simulink model "tarea"  (Simulink 7.5)
settings: Solver=ode4  StartTime=0.0  StopTime=20  FixedStep=.0001  RelTol=1e-3
values from neighbouring files (symbols this model uses):
  K1 = 3.06    [parametros.m]
  K2 = -0.7160    (= -0.716)    [parametros.m]
  L1 = 2*zo*wno-ka/(m*l)    (= 35.8260869565)    [parametros.m]
  L2 = wno^2-L1*ka/(m*l)-g/l    (= 275.117202268)    [parametros.m]
undefined symbols (not defined in the file or in its folder): G, Ka, L, M
settings Model: Creator=Lalo  LastModifiedBy=Lalo
settings OptimizationCC: ExpressionDepthLimit=128
settings DebuggingCC: UnderspecifiedInitializationDetection=Simplified  FcnCallInpInsideContextMsg=Enable All  StateNameClashWarn=none
settings CodeAppCC: CustomSymbolStrType=$N$R$M_T
settings GRTTargetCC: TargetFunctionLibrary=C89/C90 (ANSI)

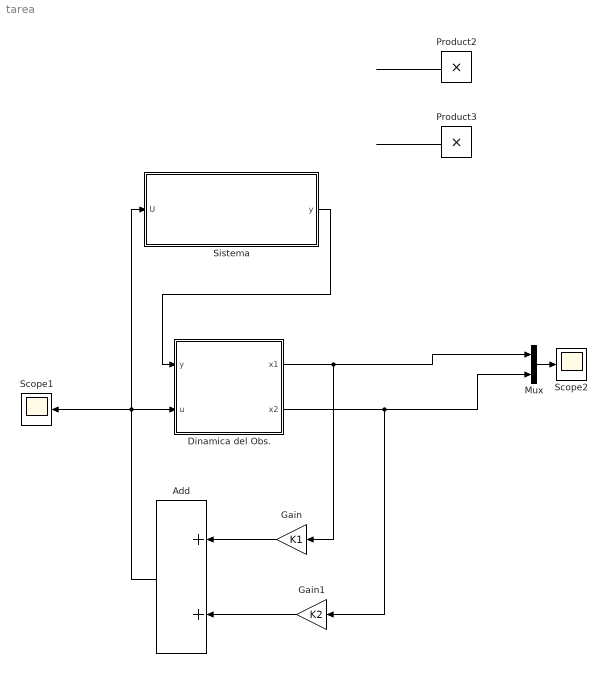
== system tarea ==
  Add : Sum
  Dinamica del Obs. : Subsystem
  Gain : Gain  Gain=K1
  Gain1 : Gain  Gain=K2
  Mux : Mux  Inputs=2
  Product2 : Product
  Product3 : Product
  Scope1 : Scope
  Scope2 : Scope
      settings: TimeRange=0.5  YMin=0  YMax=4e+75  SaveName=ScopeData2
  Sistema : Subsystem
  wires:
  Sistema/1("y ") -> Dinamica del Obs./1("y ")
  Add/1 -> Sistema/1(U), Scope1/1, Dinamica del Obs./2("u ")
  Dinamica del Obs./2("x2 ") -> Gain1/1, Mux/2
  Dinamica del Obs./1(x1) -> Gain/1, Mux/1
  Mux/1 -> Scope2/1
  ? -> Product3/2
  ? -> Product2/2
  Product2/1 -> ?
  Product3/1 -> ?
  ? -> Product2/1
  ? -> Product3/1
  Gain/1 -> Add/1
  Gain1/1 -> Add/2

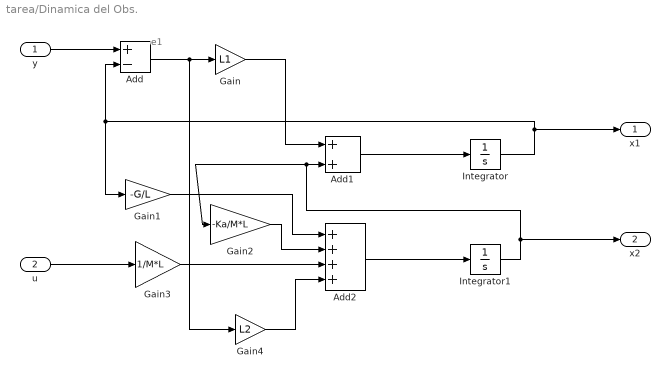
== system tarea/Dinamica del Obs. ==
  note: e1
  "y " : Inport
  "u " : Inport  Port=2
  Add : Sum  Inputs=+-
  Add1 : Sum
  Add2 : Sum  Inputs=++++
  Gain : Gain  Gain=L1
  Gain1 : Gain  Gain=-G/L
  Gain2 : Gain  Gain=-Ka/M*L
  Gain3 : Gain  Gain=1/M*L
  Gain4 : Gain  Gain=L2
  Integrator : Integrator
  Integrator1 : Integrator
  x1 : Outport
  "x2 " : Outport  Port=2
  wires:
  "u "/1 -> Gain3/1
  Gain4/1 -> Add2/4
  Integrator/1 -> x1/1, Add/2, Gain1/1
  Gain/1 -> Add1/1
  Gain3/1 -> Add2/3
  Gain2/1 -> Add2/2
  Add1/1 -> Integrator/1
  Add2/1 -> Integrator1/1
  Integrator1/1 -> "x2 "/1, Add1/2, Gain2/1
  Add/1 -> Gain4/1, Gain/1
  Gain1/1 -> Add2/1
  "y "/1 -> Add/1

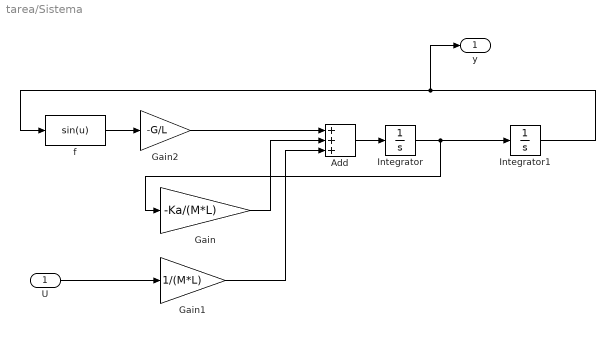
== system tarea/Sistema ==
  U : Inport
  Add : Sum  Inputs=+++
  Gain : Gain  Gain=-Ka/(M*L)
  Gain1 : Gain  Gain=1/(M*L)
  Gain2 : Gain  Gain=-G/L
  Integrator : Integrator
  Integrator1 : Integrator  InitialCondition=pi/2
  "f " : Fcn  Expr=sin(u)
  "y " : Outport
  wires:
  "f "/1 -> Gain2/1
  Integrator1/1 -> "y "/1, "f "/1
  U/1 -> Gain1/1
  Gain/1 -> Add/2
  Gain1/1 -> Add/3
  Add/1 -> Integrator/1
  Integrator/1 -> Gain/1, Integrator1/1
  Gain2/1 -> Add/1
